simulink model "simu_heli"  (R2021a)
settings: Solver=VariableStepAuto  StartTime=0.0  StopTime=30  RelTol=1e-3
values from neighbouring files (symbols this model uses):
  A_mimo = [0 0 1 0; 0 0 0 1; -den_pitch(3) 0 -den_pitch(2) 0; 0 0 0 -den_yaw(2)]    [modelos.m]
  B_mimo = [pitchFCC.b(1) 0; num_combi(2) 0; pitchFCC.b(2) 0; 0 num_yaw(3)]    [modelos.m]
  C_mimo = [1 0 0 0; 0 1 0 0]    [modelos.m]
  K = Ks(:, 1:4)    [modelos.m]
  K_lqr = Kss(:, 1:4)    [modelos.m]
  Ki = -Ks(:, 5:6)    [modelos.m]
  Ki_lqr = -Kss(:, 5:6)    [modelos.m]
undefined symbols (not defined in the file or in its folder): sigbuilder_block
settings Model: Creator=Esteban Arias  LastModifiedBy=Esteban Arias

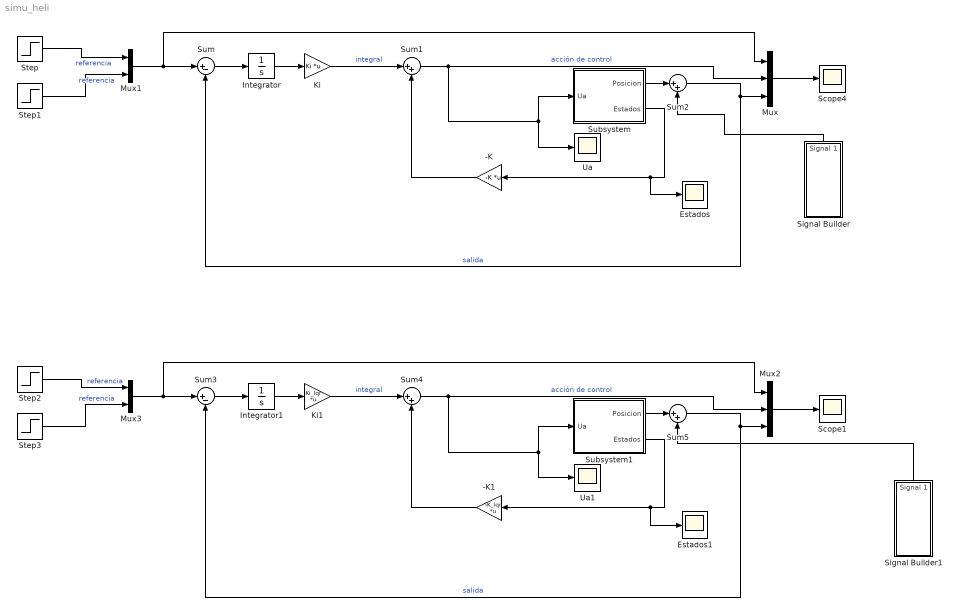
== system simu_heli ==
  -K : Gain  Gain=-K  Multiplication=Matrix(K*u)
  -K1 : Gain  Gain=-K_lqr  Multiplication=Matrix(K*u)
  Estados : Scope
  Estados1 : Scope
  Integrator : Integrator
  Integrator1 : Integrator
  Ki : Gain  Gain=Ki  Multiplication=Matrix(K*u)
  Ki1 : Gain  Gain=Ki_lqr  Multiplication=Matrix(K*u)
  Mux : Mux  Inputs=3
  Mux1 : Mux  Inputs=2
  Mux2 : Mux  Inputs=3
  Mux3 : Mux  Inputs=2
  Scope1 : Scope
  Scope4 : Scope
  Signal Builder : Subsystem  Tag=STV Subsys  LoadFcn=sigbuilder_block('load');  StartFcn=sigbuilder_block('start');  StopFcn=sigbuilder_block('stop');  ClipboardFcn=sigbuilder_block('clipboard');  mask(Sigbuilder block){tuvar=[0:10]}
      mask help: Simulink:masks:SigbuilderBlock_MD
      mask init:
      | if ~strcmp(get_param(bdroot(gcbh),'SimulationStatus'),'stopped') tuvar = sigbuilder_block('maskInit'); end
      settings: CopyFcn=sigbuilder_block('copy');  DeleteFcn=sigbuilder_block('delete');  ModelCloseFcn=sigbuilder_block('modelClose');  PreSaveFcn=sigbuilder_block('preSave');  PauseFcn=sigbuilder_block('pause');  ContinueFcn=sigbuilder_block('continue');  NameChangeFcn=sigbuilder_block('namechange');  OpenFcn=sigbuilder_block('open',[334.8 88.8 550.8 400.2 ]);  CloseFcn=sigbuilder_block('close');
      mask Display: plot(0, 0, 100, 100,[2, 2, 32, 32, 2], [68, 8, 8, 68, 68],[32, 2], [38, 38], [32, 19, 2],[53, 60, 44], [32, 17, 17, 2],[16, 16, 31, 31]);txt = getActiveGroup(gcbh);text(2, 100, txt,'verticalAlignment', 'top');
  Signal Builder1 : Subsystem  Tag=STV Subsys  LoadFcn=sigbuilder_block('load');  StartFcn=sigbuilder_block('start');  StopFcn=sigbuilder_block('stop');  ClipboardFcn=sigbuilder_block('clipboard');  mask(Sigbuilder block){tuvar=[0:10]}
      mask help: Simulink:masks:SigbuilderBlock_MD
      mask init:
      | if ~strcmp(get_param(bdroot(gcbh),'SimulationStatus'),'stopped') tuvar = sigbuilder_block('maskInit'); end
      settings: CopyFcn=sigbuilder_block('copy');  DeleteFcn=sigbuilder_block('delete');  ModelCloseFcn=sigbuilder_block('modelClose');  PreSaveFcn=sigbuilder_block('preSave');  PauseFcn=sigbuilder_block('pause');  ContinueFcn=sigbuilder_block('continue');  NameChangeFcn=sigbuilder_block('namechange');  OpenFcn=sigbuilder_block('open',[334.8 88.8 550.8 400.2 ]);  CloseFcn=sigbuilder_block('close');
      mask Display: plot(0, 0, 100, 100,[2, 2, 32, 32, 2], [68, 8, 8, 68, 68],[32, 2], [38, 38], [32, 19, 2],[53, 60, 44], [32, 17, 17, 2],[16, 16, 31, 31]);txt = getActiveGroup(gcbh);text(2, 100, txt,'verticalAlignment', 'top');
  Step : Step  Time=0  After=0.583  SampleTime=0
  Step1 : Step  Time=0  After=0  SampleTime=0
  Step2 : Step  Time=0  After=0.583  SampleTime=0
  Step3 : Step  Time=0  After=0  SampleTime=0
  Subsystem : Subsystem
  Subsystem1 : Subsystem
  Sum : Sum  Inputs=|+-
  Sum{1..2,4..5} (4 alike) : Sum  Inputs=|++
  Sum3 : Sum  Inputs=|+-
  Ua : Scope
  Ua1 : Scope
  wires:
  Sum2/1 -> Mux/3, Sum/2  "salida"
  Subsystem/1(Posicion) -> Sum2/1
  Subsystem/2(Estados) -> Estados/1, -K/1
  Mux/1 -> Scope4/1
  -K/1 -> Sum1/2
  Ki/1 -> Sum1/1  "integral"
  Sum/1 -> Integrator/1
  Sum1/1 -> Ua/1, Subsystem/1(Ua), Mux/2  "acción de control"
  Integrator/1 -> Ki/1
  Mux1/1 -> Mux/1, Sum/1
  Step/1 -> Mux1/1  "referencia"
  Step1/1 -> Mux1/2  "referencia"
  Step3/1 -> Mux3/2  "referencia"
  Mux3/1 -> Mux2/1, Sum3/1
  Integrator1/1 -> Ki1/1
  Sum3/1 -> Integrator1/1
  Ki1/1 -> Sum4/1  "integral"
  Sum4/1 -> Ua1/1, Subsystem1/1(Ua), Mux2/2  "acción de control"
  -K1/1 -> Sum4/2
  Mux2/1 -> Scope1/1
  Step2/1 -> Mux3/1  "referencia"
  Subsystem1/2(Estados) -> Estados1/1, -K1/1
  Signal Builder1/1(Signal 1) -> Sum5/2
  Sum5/1 -> Mux2/3, Sum3/2  "salida"
  Subsystem1/1(Posicion) -> Sum5/1
  Signal Builder/1(Signal 1) -> Sum2/2

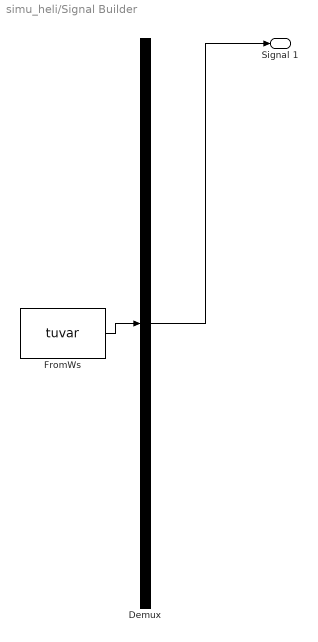
== system simu_heli/Signal Builder ==
  Demux : Demux  Tag=STV Demux  Outputs=1
      settings: DisplayOption=none
  FromWs : FromWorkspace  Tag=STV FromWs  VariableName=tuvar
      SigBuilderData=|
      | common.afterFinalStr = 'Extrapolate'
      | common.sampleTime = 0
      | dataSet.timeRange = [0 30]
      | dataSet.name = 'Group 1'
      | sbobj.Groups.Name = 'Group 1'
      | sbobj.Groups.Signals.Name = 'Signal 1'
      | sbobj.Groups.Signals.XData = [0 15 16 19 20 30]
      | sbobj.Groups.Signals.YData = [0 0 0.05 0.05 0 0]
      | sbobj.Groups.TimeRange = [0 30]
  Signal 1 : Outport  Tag=STV Outport
  wires:
  Demux/1 -> Signal 1/1
  FromWs/1 -> Demux/1

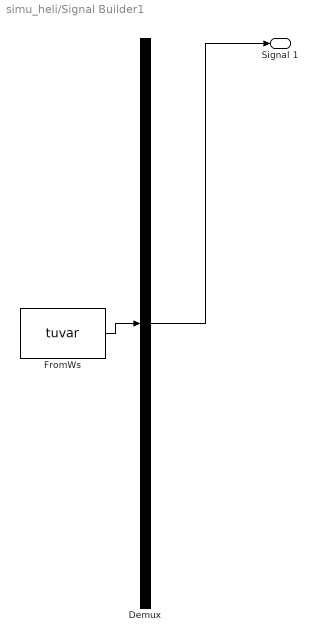
== system simu_heli/Signal Builder1 ==
  Demux : Demux  Tag=STV Demux  Outputs=1
      settings: DisplayOption=none
  FromWs : FromWorkspace  Tag=STV FromWs  VariableName=tuvar
      SigBuilderData=|
      | common.afterFinalStr = 'Extrapolate'
      | common.sampleTime = 0
      | dataSet.timeRange = [0 30]
      | dataSet.name = 'Group 1'
      | sbobj.Groups.Name = 'Group 1'
      | sbobj.Groups.Signals.Name = 'Signal 1'
      | sbobj.Groups.Signals.XData = [0 15 16 19 20 30]
      | sbobj.Groups.Signals.YData = [0 0 0.05 0.05 0 0]
      | sbobj.Groups.TimeRange = [0 30]
  Signal 1 : Outport  Tag=STV Outport
  wires:
  Demux/1 -> Signal 1/1
  FromWs/1 -> Demux/1

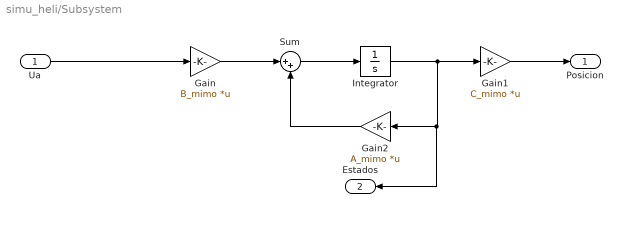
== system simu_heli/Subsystem ==
  Ua : Inport
  Gain : Gain  Gain=B_mimo  Multiplication=Matrix(K*u)
  Gain1 : Gain  Gain=C_mimo  Multiplication=Matrix(K*u)
  Gain2 : Gain  Gain=A_mimo  Multiplication=Matrix(K*u)
  Integrator : Integrator
  Sum : Sum  Inputs=|++
  Posicion : Outport
  Estados : Outport  Port=2
  wires:
  Gain/1 -> Sum/1
  Integrator/1 -> Estados/1, Gain2/1, Gain1/1
  Sum/1 -> Integrator/1
  Gain2/1 -> Sum/2
  Gain1/1 -> Posicion/1
  Ua/1 -> Gain/1

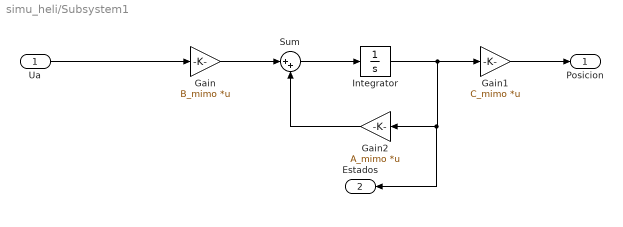
== system simu_heli/Subsystem1 ==
  Ua : Inport
  Gain : Gain  Gain=B_mimo  Multiplication=Matrix(K*u)
  Gain1 : Gain  Gain=C_mimo  Multiplication=Matrix(K*u)
  Gain2 : Gain  Gain=A_mimo  Multiplication=Matrix(K*u)
  Integrator : Integrator
  Sum : Sum  Inputs=|++
  Posicion : Outport
  Estados : Outport  Port=2
  wires:
  Gain/1 -> Sum/1
  Integrator/1 -> Estados/1, Gain2/1, Gain1/1
  Sum/1 -> Integrator/1
  Gain2/1 -> Sum/2
  Gain1/1 -> Posicion/1
  Ua/1 -> Gain/1
